simulink model "controller"  (Simulink 8.4)
settings: Solver=FixedStepDiscrete  StartTime=0.0  StopTime=inf  FixedStep=Ts  RelTol=1e-3
InitFcn:
  | initControllerDemoCodycoY1;
values from neighbouring files (symbols this model uses):
  desiredHandForces = [ 0 0 5 0 0 5]'    [initControllerDemoCodycoY1.m]
  kH = [  70    0   0 4]    [initControllerDemoCodycoY1.m]
  kImp = [kImpTorso,kImpArms,kImpArms,kImpLegs,kImpLegs]    [initControllerDemoCodycoY1.m]
  qFinHands = [ -30 20 0 40  0 ... (first row only)    [initControllerDemoCodycoY1.m]
  Rf = [R, zeros(3,3); zeros(3,3), R]    [initControllerDemoCodycoY1.m]
  states = [1 2 4 8 16]    [initControllerDemoCodycoY1.m]
  threasholdHandForces = [ 0 0 2  0 0 2]'    [initControllerDemoCodycoY1.m]
  transitionLengths = [7 10 2]    [initControllerDemoCodycoY1.m]
libraries: WBCLibrary x30, simulink x2, dspsigops x2
settings Model: Creator=daniele  LastModifiedBy=pucci
settings DataIOCC: SignalLoggingSaveFormat=Dataset
settings DebuggingCC: FcnCallInpInsideContextMsg=EnableAllAsWarning

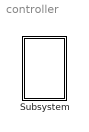
== system controller ==
  Subsystem : Subsystem  mask{robotName='iCubGenova01', Ts=0.01, localName='dynamicBalancing'}
      mask prompts: robotName "robot name"; localName "module name"

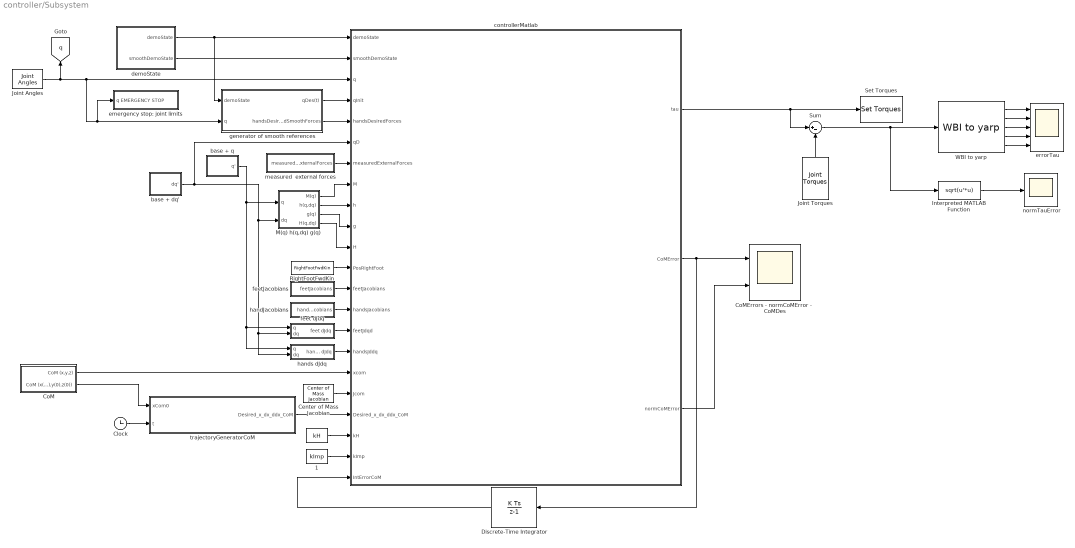
== system controller/Subsystem ==
  "    " : Constant  Value=kH
  "    1" : Constant  Value=kImp
  Center of Mass Jacobian : WBCLibrary/wholeBodyModel/Jacobians/Center of Mass Jacobian  robotName=robotName  localName=localName
  Clock : Clock
  "CoM " : Subsystem
  "CoMErrors - normCoMError -   CoMDes " : Scope  NumInputPorts=2
      settings: ShowLegends=on  TimeRange=35  YMin=-0.1~0  YMax=0.04000000000000001~0.007  SaveName=CoMErrors
  Discrete-Time Integrator : DiscreteIntegrator  InitialCondition=[0 0 0]  SampleTime=Ts
  Interpreted MATLAB Function : MATLABFcn  MATLABFcn=sqrt(u'*u)
  Joint Angles : WBCLibrary/wholeBodyStates/Joint Angles  robotName=robotName  localName=localName
  Joint Torques : WBCLibrary/wholeBodyStates/Joint Torques  robotName=robotName  localName=localName
  M(q) h(q,dq) g(q) : Subsystem
  RightFootFwdKin : WBCLibrary/wholeBodyModel/Forward Kinematics/RightFootFwdKin  robotName=robotName  localName=localName
  Set Torques : WBCLibrary/wholeBodyActuators/Set Torques  val=6  robotName=robotName  localName=localName
  Sum : Sum  Inputs=|+-
  WBI to yarp : WBCLibrary/Utilities/WBI to yarp
  base + dq' : Subsystem
  base + q : Subsystem
  controllerMatlab : MATLAB Function  TreatAsAtomicUnit=on
  demoState : Subsystem
  emergency stop: joint limits : Subsystem
  errorTau : Scope  NumInputPorts=5
      settings: TimeRange=20  YMin=-12~-5~-5~-5~-5  YMax=6~5~5~5~5
  feet dJdq : Subsystem
  feetJacobians : Subsystem
  generator of smooth references : Subsystem
  handJacobians : Subsystem
  hands dJdq : Subsystem
  measured  external forces : Subsystem
  normTauError : Scope
      settings: TimeRange=80  YMin=0  YMax=60  SaveName=normTauError
  trajectoryGeneratorCoM : MATLAB Function  TreatAsAtomicUnit=on
  tag scope: q=global
  wires:
  "    "/1 -> controllerMatlab/20(kH)
  trajectoryGeneratorCoM/1(Desired_x_dx_ddx_CoM) -> controllerMatlab/19(Desired_x_dx_ddx_CoM)
  Clock/1 -> trajectoryGeneratorCoM/2(t)
  "CoM "/2(CoM (x(0),y(0),z(0))) -> trajectoryGeneratorCoM/1(xCom0)
  RightFootFwdKin/1 -> controllerMatlab/12(PosRightFoot)
  Discrete-Time Integrator/1 -> controllerMatlab/22(IntErrorCoM)
  base + q/1(q') -> hands dJdq/1(q), feet dJdq/1(q), M(q) h(q,dq) g(q)/1(q)
  base + dq'/1(dq') -> controllerMatlab/6(qD), hands dJdq/2(dq), feet dJdq/2(dq), M(q) h(q,dq) g(q)/2(dq)
  Joint Angles/1 -> [q], generator of smooth references/2(q), emergency stop: joint limits/1(q EMERGENCY STOP), controllerMatlab/3(q)
  controllerMatlab/2(CoMError) -> Discrete-Time Integrator/1, "CoMErrors - normCoMError -   CoMDes "/1
  controllerMatlab/3(normCoMError) -> "CoMErrors - normCoMError -   CoMDes "/2
  "    1"/1 -> controllerMatlab/21(kImp)
  measured  external forces/1(measuredExternalForces) -> controllerMatlab/7(measuredExternalForces)
  Joint Torques/1 -> Sum/2
  Interpreted MATLAB Function/1 -> normTauError/1
  Sum/1 -> WBI to yarp/1, Interpreted MATLAB Function/1
  WBI to yarp/1 -> errorTau/1
  WBI to yarp/2 -> errorTau/2
  WBI to yarp/3 -> errorTau/3
  WBI to yarp/4 -> errorTau/4
  WBI to yarp/5 -> errorTau/5
  M(q) h(q,dq) g(q)/1(M(q)) -> controllerMatlab/8(M)
  M(q) h(q,dq) g(q)/2(h(q,dq)) -> controllerMatlab/9(h)
  M(q) h(q,dq) g(q)/3(g(q)) -> controllerMatlab/10(g)
  "CoM "/1(CoM (x,y,z)) -> controllerMatlab/17(xcom)
  M(q) h(q,dq) g(q)/4(H(q,dq)) -> controllerMatlab/11(H)
  Center of Mass Jacobian/1 -> controllerMatlab/18(Jcom)
  feetJacobians/1(feetJacobians) -> controllerMatlab/13(feetJacobians)
  handJacobians/1(handJacobians) -> controllerMatlab/14(handsJacobians)
  feet dJdq/1(feet dJdq) -> controllerMatlab/15(feetJdqd)
  hands dJdq/1(hands dJdq) -> controllerMatlab/16(handsJddq)
  generator of smooth references/1(qDes(t)) -> controllerMatlab/4(qInit)
  generator of smooth references/2(handsDesiredSmoothForces) -> controllerMatlab/5(handsDesiredForces)
  demoState/2(smoothDemoState) -> controllerMatlab/2(smoothDemoState)
  demoState/1(demoState) -> controllerMatlab/1(demoState), generator of smooth references/1(demoState)
  controllerMatlab/1(tau) -> Set Torques/1, Sum/1

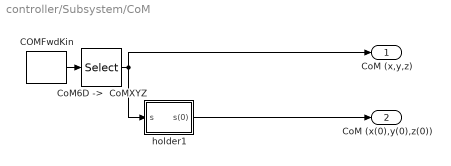
== system controller/Subsystem/CoM  ==
  "COMFwdKin " : WBCLibrary/wholeBodyModel/Forward Kinematics/COMFwdKin   robotName=robotName  localName=localName
  "CoM6D ->  CoMXYZ" : Selector  InputPortWidth=7  Indices=[1 2 3]
  holder1 : Subsystem
  CoM (x,y,z) : Outport
  CoM (x(0),y(0),z(0)) : Outport  Port=2
  wires:
  "COMFwdKin "/1 -> "CoM6D ->  CoMXYZ"/1
  "CoM6D ->  CoMXYZ"/1 -> holder1/1(s), CoM (x,y,z)/1
  holder1/1(s(0)) -> CoM (x(0),y(0),z(0))/1

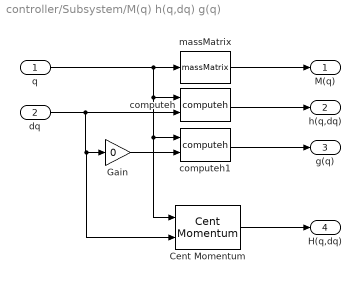
== system controller/Subsystem/M(q) h(q,dq) g(q) ==
  q : Inport
  dq : Inport  Port=2
  Cent Momentum : WBCLibrary/wholeBodyModel/Dynamics/Cent Momentum  robotName=robotName  localName=localName
  Gain : Gain  Gain=0
  computeh : WBCLibrary/wholeBodyModel/Dynamics/computeh  val=7  robotname=robotName  localname=localName
  computeh1 : WBCLibrary/wholeBodyModel/Dynamics/computeh  val=7  robotname=robotName  localname=localName
  massMatrix : WBCLibrary/wholeBodyModel/Dynamics/massMatrix  val=8  robotname=robotName  localname=localName
  M(q) : Outport
  h(q,dq) : Outport  Port=2
  g(q) : Outport  Port=3
  H(q,dq) : Outport  Port=4
  wires:
  Gain/1 -> computeh1/2
  computeh1/1 -> g(q)/1
  computeh/1 -> h(q,dq)/1
  massMatrix/1 -> M(q)/1
  q/1 -> Cent Momentum/1, computeh1/1, computeh/1, massMatrix/1
  dq/1 -> Cent Momentum/2, Gain/1, computeh/2
  Cent Momentum/1 -> H(q,dq)/1

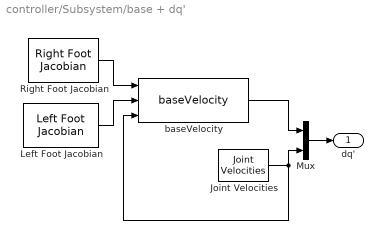
== system controller/Subsystem/base + dq' ==
  Joint Velocities : WBCLibrary/wholeBodyStates/Joint Velocities  robotName=robotName  localName=localName
  Left Foot Jacobian : WBCLibrary/wholeBodyModel/Jacobians/Left Foot Jacobian  robotName=robotName  localName=localName
  Mux : Mux  Inputs=2
  Right Foot Jacobian : WBCLibrary/wholeBodyModel/Jacobians/Right Foot Jacobian  robotName=robotName  localName=localName
  baseVelocity : WBCLibrary/Utilities/baseVelocity
  dq' : Outport
  wires:
  Left Foot Jacobian/1 -> baseVelocity/2
  Right Foot Jacobian/1 -> baseVelocity/1
  baseVelocity/1 -> Mux/1
  Joint Velocities/1 -> baseVelocity/3, Mux/2
  Mux/1 -> dq'/1

== system controller/Subsystem/base + q ==
  Constant1 : Constant  Value=zeros(16,1)
  Mux : Mux  Inputs=2
  q' : Outport
  wires:
  Mux/1 -> q'/1
  [q] -> Mux/2
  Constant1/1 -> Mux/1

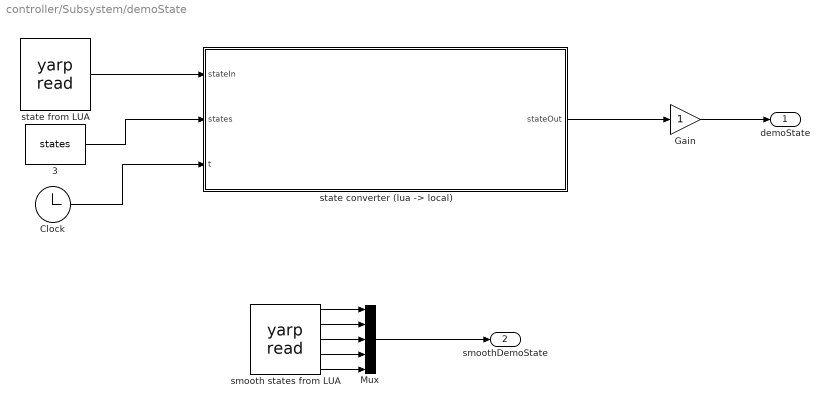
== system controller/Subsystem/demoState ==
  "    3" : Constant  Value=states
  Clock : Clock
  Gain : Gain
  Mux : Mux  Inputs=5
  smooth states from LUA : WBCLibrary/Utilities/yarp read  from='/codycoCoordinator1Y/smooth_state:o'  to='...'  num=5
  "state converter (lua -> local)" : MATLAB Function  TreatAsAtomicUnit=on
  state from LUA : WBCLibrary/Utilities/yarp read  from='/codycoCoordinator1Y/state:o'  to='...'  num=1
  demoState : Outport
  smoothDemoState : Outport  Port=2
  wires:
  Gain/1 -> demoState/1
  "    3"/1 -> "state converter (lua -> local)"/2(states)
  Clock/1 -> "state converter (lua -> local)"/3(t)
  "state converter (lua -> local)"/1(stateOut) -> Gain/1
  state from LUA/1 -> "state converter (lua -> local)"/1(stateIn)
  smooth states from LUA/1 -> Mux/1
  Mux/1 -> smoothDemoState/1
  smooth states from LUA/2 -> Mux/2
  smooth states from LUA/3 -> Mux/3
  smooth states from LUA/4 -> Mux/4
  smooth states from LUA/5 -> Mux/5

== system controller/Subsystem/emergency stop: joint limits ==
  q EMERGENCY STOP : Inport
  Assertion : Assertion
  Joint Limits1 : WBCLibrary/wholeBodyModel/Joint Limits  robotName=robotName  localName=localName
  MATLAB Function : MATLAB Function  TreatAsAtomicUnit=on
  index1 : Constant  Value=0.01  VectorParams1D=off
  wires:
  Joint Limits1/1 -> MATLAB Function/1(umin)
  Joint Limits1/2 -> MATLAB Function/2(umax)
  index1/1 -> MATLAB Function/4(tol)
  q EMERGENCY STOP/1 -> MATLAB Function/3(u)
  MATLAB Function/1(inRange) -> Assertion/1

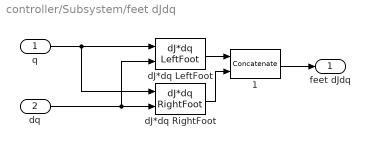
== system controller/Subsystem/feet dJdq ==
  q : Inport
  dq : Inport  Port=2
  " 1" : Concatenate  Mode=Multidimensional array
  dJ*dq LeftFoot : WBCLibrary/wholeBodyModel/Dynamics/dJ*dq LeftFoot  val=9  robotName=robotName  localName=localName
  dJ*dq RightFoot : WBCLibrary/wholeBodyModel/Dynamics/dJ*dq RightFoot  val=9  robotName=robotName  localName=localName
  feet dJdq : Outport
  wires:
  dJ*dq LeftFoot/1 -> " 1"/1
  dJ*dq RightFoot/1 -> " 1"/2
  " 1"/1 -> feet dJdq/1
  q/1 -> dJ*dq RightFoot/1, dJ*dq LeftFoot/1
  dq/1 -> dJ*dq LeftFoot/2, dJ*dq RightFoot/2

== system controller/Subsystem/feetJacobians ==
  " " : Concatenate  Mode=Multidimensional array
  Left Foot Jacobian : WBCLibrary/wholeBodyModel/Jacobians/Left Foot Jacobian  robotName=robotName  localName=localName
  Right Foot Jacobian : WBCLibrary/wholeBodyModel/Jacobians/Right Foot Jacobian  robotName=robotName  localName=localName
  feetJacobians : Outport
  wires:
  Left Foot Jacobian/1 -> " "/1
  Right Foot Jacobian/1 -> " "/2
  " "/1 -> feetJacobians/1

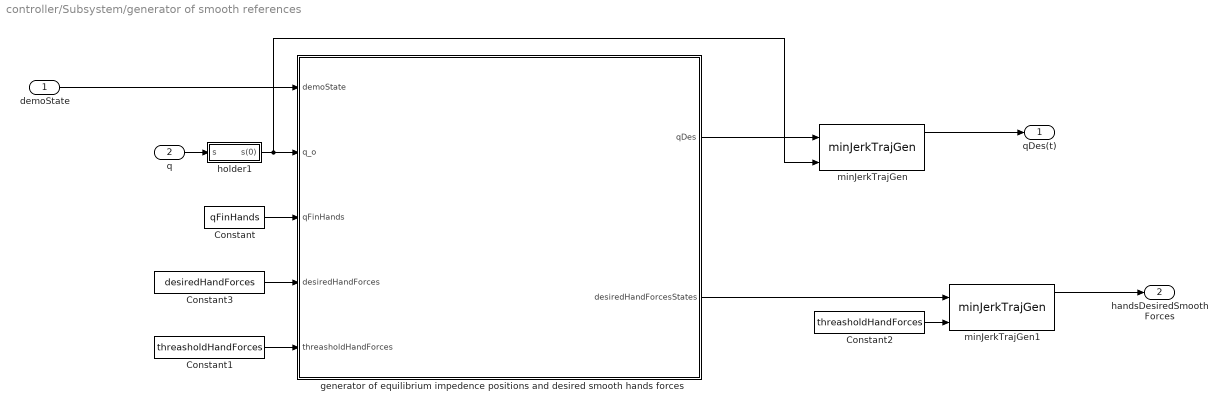
== system controller/Subsystem/generator of smooth references ==
  demoState : Inport
  q : Inport  Port=2
  Constant : Constant  Value=qFinHands
  Constant1 : Constant  Value=threasholdHandForces
  Constant2 : Constant  Value=threasholdHandForces
  Constant3 : Constant  Value=desiredHandForces
  generator of equilibrium impedence positions and desired smooth hands forces : MATLAB Function  TreatAsAtomicUnit=on
  holder1 : Subsystem
  minJerkTrajGen : WBCLibrary/Utilities/minJerkTrajGen  dim=25  Ts=Ts  Tt=transitionLengths(1)
  minJerkTrajGen1 : WBCLibrary/Utilities/minJerkTrajGen  dim=6  Ts=Ts  Tt=transitionLengths(2)
  qDes(t) : Outport
  handsDesiredSmoothForces : Outport  Port=2
  wires:
  q/1 -> holder1/1(s)
  Constant/1 -> generator of equilibrium impedence positions and desired smooth hands forces/3(qFinHands)
  holder1/1(s(0)) -> minJerkTrajGen/2, generator of equilibrium impedence positions and desired smooth hands forces/2(q_o)
  demoState/1 -> generator of equilibrium impedence positions and desired smooth hands forces/1(demoState)
  Constant3/1 -> generator of equilibrium impedence positions and desired smooth hands forces/4(desiredHandForces)
  Constant1/1 -> generator of equilibrium impedence positions and desired smooth hands forces/5(threasholdHandForces)
  generator of equilibrium impedence positions and desired smooth hands forces/1(qDes) -> minJerkTrajGen/1
  minJerkTrajGen/1 -> qDes(t)/1
  generator of equilibrium impedence positions and desired smooth hands forces/2(desiredHandForcesStates) -> minJerkTrajGen1/1
  Constant2/1 -> minJerkTrajGen1/2
  minJerkTrajGen1/1 -> handsDesiredSmoothForces/1

== system controller/Subsystem/handJacobians ==
  " " : Concatenate  Mode=Multidimensional array
  Left Hand Jacobian : WBCLibrary/wholeBodyModel/Jacobians/Left Hand Jacobian  robotName=robotName  localName=localName
  Right Hand Jacobian : WBCLibrary/wholeBodyModel/Jacobians/Right Hand Jacobian  robotName=robotName  localName=localName
  handJacobians : Outport
  wires:
  " "/1 -> handJacobians/1
  Left Hand Jacobian/1 -> " "/1
  Right Hand Jacobian/1 -> " "/2

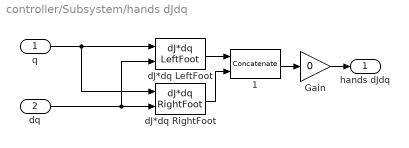
== system controller/Subsystem/hands dJdq ==
  q : Inport
  dq : Inport  Port=2
  " 1" : Concatenate  Mode=Multidimensional array
  Gain : Gain  Gain=0
  dJ*dq LeftFoot : WBCLibrary/wholeBodyModel/Dynamics/dJ*dq LeftFoot  val=9  robotName=robotName  localName=localName
  dJ*dq RightFoot : WBCLibrary/wholeBodyModel/Dynamics/dJ*dq RightFoot  val=9  robotName=robotName  localName=localName
  hands dJdq : Outport
  wires:
  dJ*dq LeftFoot/1 -> " 1"/1
  dJ*dq RightFoot/1 -> " 1"/2
  " 1"/1 -> Gain/1
  q/1 -> dJ*dq RightFoot/1, dJ*dq LeftFoot/1
  dq/1 -> dJ*dq LeftFoot/2, dJ*dq RightFoot/2
  Gain/1 -> hands dJdq/1

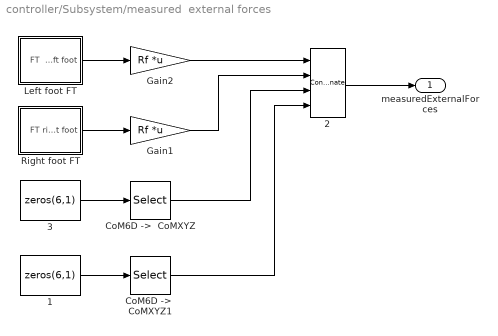
== system controller/Subsystem/measured  external forces ==
  "    1" : Constant  Value=zeros(6,1)
  "    3" : Constant  Value=zeros(6,1)
  " 2" : Concatenate  NumInputs=4  Mode=Multidimensional array
  "CoM6D ->  CoMXYZ" : Selector  InputPortWidth=6  Indices=[1 2 3]
  "CoM6D ->  CoMXYZ1" : Selector  InputPortWidth=6  Indices=[1 2 3]
  Gain1 : Gain  Gain=Rf  Multiplication=Matrix(K*u)
  Gain2 : Gain  Gain=Rf  Multiplication=Matrix(K*u)
  Left foot FT : Subsystem
  Right foot FT : Subsystem
  measuredExternalForces : Outport
  wires:
  Right foot FT/1(FT right foot) -> Gain1/1
  Left foot FT/1(FT  left foot) -> Gain2/1
  Gain2/1 -> " 2"/1
  Gain1/1 -> " 2"/2
  " 2"/1 -> measuredExternalForces/1
  "    3"/1 -> "CoM6D ->  CoMXYZ"/1
  "    1"/1 -> "CoM6D ->  CoMXYZ1"/1
  "CoM6D ->  CoMXYZ"/1 -> " 2"/3
  "CoM6D ->  CoMXYZ1"/1 -> " 2"/4

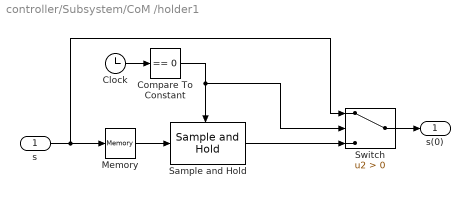
== system controller/Subsystem/CoM /holder1 ==
  s : Inport
  Clock : Clock
  Compare To Constant : simulink/Logic and Bit Operations/Compare To Constant  relop===  const=0  OutDataTypeStr=boolean
  Memory : Memory
  Sample and Hold : dspsigops/Sample and Hold  trig=Falling edge  initCond=0  latchinput=off
  Switch : Switch  Criteria=u2 > Threshold
  s(0) : Outport
  wires:
  s/1 -> Switch/1, Memory/1
  Clock/1 -> Compare To Constant/1
  Compare To Constant/1 -> Sample and Hold/Trigger, Switch/2
  Sample and Hold/1 -> Switch/3
  Switch/1 -> s(0)/1
  Memory/1 -> Sample and Hold/1

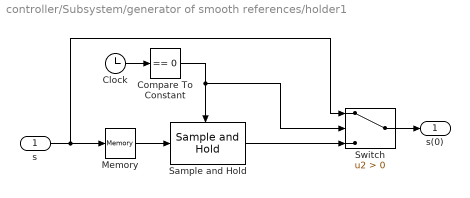
== system controller/Subsystem/generator of smooth references/holder1 ==
  s : Inport
  Clock : Clock
  Compare To Constant : simulink/Logic and Bit Operations/Compare To Constant  relop===  const=0  OutDataTypeStr=boolean
  Memory : Memory
  Sample and Hold : dspsigops/Sample and Hold  trig=Falling edge  initCond=0  latchinput=off
  Switch : Switch  Criteria=u2 > Threshold
  s(0) : Outport
  wires:
  s/1 -> Switch/1, Memory/1
  Clock/1 -> Compare To Constant/1
  Compare To Constant/1 -> Sample and Hold/Trigger, Switch/2
  Sample and Hold/1 -> Switch/3
  Switch/1 -> s(0)/1
  Memory/1 -> Sample and Hold/1

== system controller/Subsystem/measured  external forces/Left foot FT ==
  Mux : Mux  Inputs=6
  yarp read : WBCLibrary/Utilities/yarp read  from='/wholeBodyDyanmicsTree/left_leg/endEffectorWrench:o'  to='...'  num=6
  FT  left foot : Outport
  wires:
  yarp read/1 -> Mux/1
  yarp read/2 -> Mux/2
  yarp read/3 -> Mux/3
  yarp read/4 -> Mux/4
  yarp read/5 -> Mux/5
  yarp read/6 -> Mux/6
  Mux/1 -> FT  left foot/1

== system controller/Subsystem/measured  external forces/Right foot FT ==
  Mux : Mux  Inputs=6
  yarp read : WBCLibrary/Utilities/yarp read  from='/wholeBodyDyanmicsTree/right_leg/endEffectorWrench:o'  to='...'  num=6
  FT right foot : Outport
  wires:
  yarp read/1 -> Mux/1
  yarp read/2 -> Mux/2
  yarp read/3 -> Mux/3
  yarp read/4 -> Mux/4
  yarp read/5 -> Mux/5
  yarp read/6 -> Mux/6
  Mux/1 -> FT right foot/1

== matlab function Subsystem/trajectoryGeneratorCoM ==
  data: Desired_x_dx_ddx_CoM output double; xCom0 input double; t input double
function Desired_x_dx_ddx_CoM = fcn(xCom0,t)
%#codegen

e3 = [0;1;0];
A = 0.0;
f = 0.15;

xcomDes    = xCom0 + A*sin(2*pi*f*t)*e3;
% xcomDes(1) =  xcomDes(1) + 0.01;
xDcomDes   =         A*2*pi*f*cos(2*pi*f*t)*e3;
xDDcomDes  =        -A*(2*pi*f)^2*sin(2*pi*f*t)*e3;

Desired_x_dx_ddx_CoM = [xcomDes,xDcomDes,xDDcomDes];

== matlab function Subsystem/controllerMatlab ==
  data: demoState input double; smoothDemoState input double; q input double; qInit input double; handsDesiredForces input double; qD input double; measuredExternalForces input double; M input double; h input double; g input double; H input double; PosRightFoot input double; feetJacobians input double; handsJacobians input double; tau output double; feetJdqd input double; handsJddq input double; xcom input double; Jcom input double; Desired_x_dx_ddx_CoM input double; kH input double; kImp input double; CoMError output double; IntErrorCoM input double; normCoMError output double
function [tau,CoMError,normCoMError] = fcn(demoState,smoothDemoState,q,qInit,handsDesiredForces,qD, measuredExternalForces, M, h, g, H, PosRightFoot, feetJacobians, handsJacobians,feetJdqd,handsJddq, xcom,Jcom, Desired_x_dx_ddx_CoM, kH, kImp, IntErrorCoM)
%#codegen

PINV_TOL = 1e-5;
gravAcc        = 9.81;

n = 25;
St    = [zeros(6,n);eye(n,n)];

m     = M(1,1);
grav = [zeros(2,1);-m*gravAcc;zeros(3,1)];

% Definition of reference accelerations for CoM and Joints that ensure
% stabilization of desired trajectories xDcomDes and qDes 

xDcom      = Jcom(1:3,:)*qD;
xDDcomStar = Desired_x_dx_ddx_CoM(:,3) - kH(1)*(xcom - Desired_x_dx_ddx_CoM(:,1)) - kH(2)*IntErrorCoM - kH(3)*(xDcom - Desired_x_dx_ddx_CoM(:,2));

Pr =  PosRightFoot(1:3) - xcom; % Application point of the contact force on the right foot w.r.t. CoM

A  = [ eye(3),   zeros(3),eye(3), zeros(3);
      -Sf(xcom),  eye(3), Sf(Pr), eye(3) ];
pinvA = pinv(A, PINV_TOL);
  
  
HwDotDes = H(4:end);




    
HDotDes  = [ m*xDDcomStar ;
            -kH(4)*HwDotDes  ]; 

contactOnLeftHandState  = 3;
contactOnRightHandState = 4;
contactOnBothHandsState = 5;




% % if demoState == 0 || demoState == 1 %State: balancing, no hand motion
%      Jc    = [ feetJacobians;
%                zeros(6,31)];       
%      JcDqD = [ feetJdqd;
%                zeros(6,1)];
%      handsDesiredWrenches = zeros(6,1);
% % end
% 
% if demoState == 2 %State: contact on the left hand is occurred, right hand keeps moving
% 	Jc    = [ feetJacobians;
%               handsJacobians(1:3,:);
%               zeros(3,31)];       
%     JcDqD = [ feetJdqd;
%               handsJddq(1:3);
%               zeros(3,1)];
%      
%     handsDesiredWrenches = [ handsDesiredForces(1:3);
%                              zeros(3,1)];
% end
% 
% if demoState == 3 %State: contact on the right hand is occurred, left hand keeps moving
% 	Jc    = [ feetJacobians;
%               zeros(3,31);
%               handsJacobians(7:9,:);];       
%     JcDqD = [ feetJdqd;
%               zeros(3,1);
%               handsJddq(7:9)];
%      
%     handsDesiredWrenches = [ handsDesiredForces(4:6);
%                              zeros(3,1)];
% end
% 
% if demoState == 4  %State: both hands are in contact
% 	Jc    = [ feetJacobians;
%               handsJacobians(1:3,:);
%               handsJacobians(7:9,:)];       
%     JcDqD = [ feetJdqd;
%               handsJddq(1:3);
%               handsJddq(7:9)];
%      
%     handsDesiredWrenches = [ handsDesiredForces(1:3) + handsDesiredForces(4:6);
%                              zeros(3,1)];
% end  

Jc    = [ feetJacobians;
          handsJacobians(1:3,:)*(smoothDemoState(contactOnLeftHandState) + smoothDemoState(contactOnBothHandsState)) ;
          handsJacobians(7:9,:)*(smoothDemoState(contactOnRightHandState) + smoothDemoState(contactOnBothHandsState))];       
JcDqD = [feetJdqd;
         handsJddq(1:3)*(smoothDemoState(contactOnLeftHandState) + smoothDemoState(contactOnBothHandsState));
         handsJddq(7:9)*(smoothDemoState(contactOnRightHandState) + smoothDemoState(contactOnBothHandsState))*0];

    handsDesiredWrenches = [ handsDesiredForces(1:3)*(smoothDemoState(contactOnLeftHandState) + smoothDemoState(contactOnBothHandsState)) + handsDesiredForces(4:6)*(smoothDemoState(contactOnRightHandState) + smoothDemoState(contactOnBothHandsState));
                             zeros(3,1)];
     
feetDesiredWrenches = pinvA*(HDotDes-grav-handsDesiredWrenches);

desiredExternalWrench = [ feetDesiredWrenches;
                          handsDesiredForces  ];
    

Minv = inv(M);
JcMinv        = Jc*Minv;
PInv_JcMinvSt = pinv(JcMinv*St, PINV_TOL);
N0            = eye(n) - PInv_JcMinvSt*JcMinv*St;

measuredExternalWrench = desiredExternalWrench;

tau1 = PInv_JcMinvSt*(JcMinv*h - JcDqD - JcMinv*Jc'*desiredExternalWrench);
LinearizedDynamics = g(7:end)-Jc(:,7:end)'*measuredExternalWrench - kImp.*(q-qInit);% - tau1; %-diag(kDam)*N0'*qD(7:end) ;  %-kDam.*qD(7:end) 

tau0 = LinearizedDynamics;

tau = tau1 + N0*tau0;

% f = (JcMinv*Jc')^-1*(JcMinv*(h-[zeros(6,1);tau])-JcDqD);

CoMError    = xcom - Desired_x_dx_ddx_CoM(:,1);
normCoMError  = norm(CoMError);

== matlab function Subsystem/generator of smooth references/generator of equilibrium impedence positions and desired smooth hands forces ==
  data: demoState input double; q_o input double; qFinHands input double; qDes output double; desiredHandForces input double; desiredHandForcesStates output double; threasholdHandForces input double
function [qDes,desiredHandForcesStates] = impedenceEquilibriumPositionGenerator(demoState,q_o,qFinHands,desiredHandForces,threasholdHandForces)
%#codegen
    
    desiredHandForcesStates = threasholdHandForces;
        
    qDes = q_o;
    qDes(4:8) = qFinHands(1,:);%qFinHands(2,:)];
    qDes(9:13) = qFinHands(2,:);%qFinHands(2,:)];
    

    if demoState == 0 %State: balancing, no hand motion
        qDes = q_o;
    end

    if demoState == 1 %State: seeking contacts, both hands are moving
    end

    if demoState == 2 %State: contact on the left hand is occurred, right hand keeps moving
        desiredHandForcesStates(1:3) = desiredHandForces(1:3);
    end

    if demoState == 3 %State: contact on the right hand is occurred, left hand keeps moving
        desiredHandForcesStates(4:6) = desiredHandForces(4:6);
    end

    if demoState == 4  %State: both hands are in contact
        desiredHandForcesStates = desiredHandForces;
    end  

end

== matlab function Subsystem/emergency stop: joint limits/MATLAB Function ==
  data: umin input double; umax input double; u input double; inRange output double; tol input double
function inRange = checkRange(umin, umax, u, tol)
%#codegen

res = u < umin + tol | u > umax - tol;
res = sum(res);
if res==0
    inRange = 1;
else
    inRange = 0;
    u < umin + tol | u > umax - tol
end

== matlab function Subsystem/demoState/state converter (lua -> local) ==
  data: stateIn input double; stateOut output double; states input double; t input double
function stateOut = convertingDemoStatesIntoStrings(stateIn,states,t)
%#codegen
 
stateOut = 0; 
if stateIn == states(1)
    stateOut = 0;
end

if stateIn == states(2)
    stateOut = 1;
end

if stateIn == states(3)
    stateOut = 2;
end

if stateIn == states(4)
    stateOut = 3;
end

if stateIn == states(5)
    stateOut = 4; 
end

% T = 5;
% if  (0 <= t  && t < T ) 
%     stateOut = 0;
% end
% 
% if  (T <= t && t < 2*T ) 
%     stateOut = 1;
% end
% 
% if  (2*T <= t && t < 3*T ) 
%     stateOut = 0;
% end
% 
% if  (3*T <= t && t < 4*T ) 
%     stateOut = 1;
% end
% 
% if  (4*T <= t && t < 5*T)
%     stateOut = 4;
% end
% 
% if (5*T <= t && t < 6*T)
%     stateOut = 2;
% end
% 
% if  (6*T <= t && t < 7*T)
%     stateOut = 4;
% end
% 
% if (7*T <= t  && t < 8*T)
%     stateOut = 3;
% end
% 
% if  (8*T <= t  && t < 9*T ) 
%     stateOut = 4;
% end
% 
% if  (9*T <= t && t < 10*T ) 
%     stateOut = 0;
% end
% 
% if  (10*T <= t && t < 11*T ) 
%     stateOut = 1;
% end
% 
% if  (11*T <= t  && t < 12*T ) 
%     stateOut = 2;
% end
% 
% if (12*T <= t  && t < 13*T)
%     stateOut = 4;
% end
% 
% if  (13*T <= t  && t < 14*T ) 
%     stateOut = 0;
% end
% 
% if  (14*T <= t && t < 15*T ) 
%     stateOut = 1;
% end
% 
% if  (15*T <= t  && t < 16*T ) 
%     stateOut = 3;
% end
% 
% if (16*T <= t  && t < 17*T)
%     stateOut = 4;
% end
% 
% if  (17*T <= t  && t < 18*T ) 
%     stateOut = 0;
% end
% 
% if (18*T <= t  && t < 19*T)
%     stateOut = 4;
% end
% 
% if  (19*T <= t  ) 
%     stateOut = 0;
% end
% 
%
